simulink model "mech_sticky_box"  (Simulink 7.1)
settings: Solver=ode23t  StartTime=0.0  StopTime=10  RelTol=1e-4  AbsTol=1e-7
libraries: mblibv1 x11, mech_friction x2
Description:
  | Sticky Sliding Boxes
  | 
  | A box sliding on top of another box with sticky friction.
  | 
  | This model demonstrates the use of a stiction actuator. It adds stiction between three boxes on their contacting surfaces. The bottom box is motion-actuated. The velocity plots show periods of zero velocity, indicating locking.
settings Model: Creator=arnav  LastModifiedBy=batserve  ExtModeAutoUpdateStatusClock=off
settings SolverCC: MaxConsecutiveMinStep=10  SolverResetMethod=Robust
settings DataIOCC: OutputOption=SpecifiedOutputTimes  OutputTimes=linspace(0,10,200)  Refine=5
settings OptimizationCC: InlineInvariantSignals=on  BufferReusableBoundary=off
settings DebuggingCC: AlgebraicLoopMsg=none  SaveWithParameterizedLinksMsg=none  SignalResolutionControl=TryResolveAllWithWarning  SolverPrmCheckMsg=none  MultiTaskDSMMsg=warning  MultiTaskCondExecSysMsg=none  SigSpecEnsureSampleTimeMsg=none  UnconnectedInputMsg=none  UnconnectedOutputMsg=none  BusObjectLabelMismatch=none  StrictBusMsg=None
settings HardwareCC: TargetBitPerLong=64  TargetEndianess=LittleEndian  TargetWordSize=64  TargetHWDeviceType=MATLAB Host  ProdEqTarget=off
settings RTWCC: SystemTargetFile=rsim.tlc  TemplateMakefile=rsim_default_tmf  Description=Rapid Simulation Target  ProcessScript=rsim_make_rtw_hook  IncludeERTFirstTime=on
settings RSimTargetCC: TargetFcnLib=ansi_tfl_tmw.mat  TargetFunctionLibrary=ANSI_C  IsPILTarget=off  EnableShiftOperators=on  PortableWordSizes=off
settings SimMechanicsCC: WarnOnRedundantConstraints=off  VisOnUpdateDiagram=on  VisDuringSimulation=on  VisConfigFile=mech_sticky_box.mat

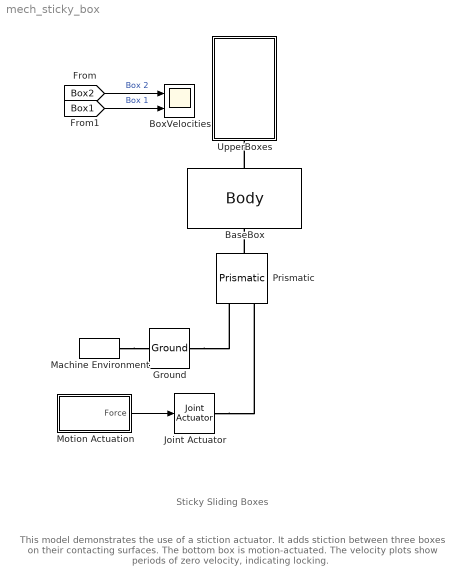
== system mech_sticky_box ==
  note: This model demonstrates the use of a stiction actuator.
      | It adds stiction between three boxes on their contacting surfaces.
      | The bottom box is motion-actuated. The velocity plots show periods
      | of zero velocity, indicating locking.
  note: Sticky Sliding Boxes
  BaseBox : mblibv1/Bodies/Body  Orientation=up  DialogController=MECH.DynMechDlgSource  PhysicalDomain=mechanical  SubClassName=Unknown  LeftPortType=workingframe  RightPortType=workingframe  LConnTagsString=CS1  RConnTagsString=CS2  DialogClass=MechanicalBodyBlock  Mass=1  MassUnits=kg  InertiaUnits=kg*m^2  Inertia=[1 0 0;0 1.9 0;0 0 1]  Shape=Cylinder  ShapeDims=[1 1]  ShapeUnits=m  ShapeUse=false  Density=1  DensityUnits=kg/m^3  DensityUse=false  GraphicsMode=1  BodyColor=[0.5 0.5 0.5]  GraphicsObj=[]  AttachedToCS=1  CG=Left$CG$[0 0.5 0]$CS1$CS1$m$[0 0 0]$Euler X-Y-Z$deg$WORLD$false  WorkingFrames=Left$CS1$[0 0 0]$ADJOINING$ADJOINING$m$[0 0 0]$Euler X-Y-Z$deg$WORLD$true#Right$CS2$[0 1 0]$CS1$CS1$m$[0 0 0]$Euler X-Y-Z$deg$WORLD$true#Right$CS3$[-2 0 2]$CS1$CS1$m$[0 0 0]$Euler X-Y-Z$deg$WORLD$false#Right$CS7$[0 1 0]$CS3$CS3$m$[0 0 0]$Euler X-Y-Z$deg$WORLD$false#Right$CS4$[2 0 2]$CS1$CS1$m$[0 0 0]$Euler X-Y-Z$deg$WORLD$false#Right$CS8$[0 1 0]$CS4$CS4$m$[0 0 0]$Euler X-Y-Z$deg$WORLD$false#Right$CS5$[2 0 -2]$CS1$CS1$m$[0 0 0]$Euler X-Y-Z$deg$WORLD$false#Right$CS9$[0 1 0]$CS5$CS5$m$[0 0 0]$Euler X-Y-Z$deg$WORLD$false#Right$CS6$[-2 0 -2]$CS1$CS1$m$[0 0 0]$Euler X-Y-Z$deg$WORLD$false#Right$CS10$[0 1 0]$CS6$CS6$m$[0 0 0]$Euler X-Y-Z$deg$WORLD$false  CGPos=[0 0.5 0]  CGRot=[0 0 0]  CS0Pos=[]  CS0Rot=[]  CS1Pos=[0 0 0]  CS1Rot=[0 0 0]  CS2Pos=[0 1 0]  CS2Rot=[0 0 0]  CS3Pos=[-2 0 2]  CS3Rot=[0 0 0]  CS4Pos=[2 0 2]  CS4Rot=[0 0 0]  CS5Pos=[2 0 -2]  CS5Rot=[0 0 0]  CS6Pos=[-2 0 -2]  CS6Rot=[0 0 0]  CS7Pos=[0 1 0]  CS7Rot=[0 0 0]  CS8Pos=[0 1 0]  CS8Rot=[0 0 0]  CS9Pos=[0 1 0]  CS9Rot=[0 0 0]  CS10Pos=[0 1 0]  CS10Rot=[0 0 0]  CS11Pos=[]  CS11Rot=[]  CS12Pos=[]  CS12Rot=[]  CS13Pos=[]  CS13Rot=[]  CS14Pos=[]  CS14Rot=[]  CS15Pos=[]  CS15Rot=[]  CS16Pos=[]  CS16Rot=[]  CS17Pos=[]  CS17Rot=[]  CS18Pos=[]  CS18Rot=[]  CS19Pos=[]  CS19Rot=[]  CS20Pos=[]  CS20Rot=[]
  BoxVelocities : Scope  NumInputPorts=2
      settings: TimeRange=10  YMin=-0.4~-1.5  YMax=0.4~1.5
  Ground : mblibv1/Bodies/Ground  DialogController=MECH.DynMechDlgSource  SystemSampleTime=-1  LeftPortType=env  RightPortType=workingframe  PhysicalDomain=Mechanical  DialogClass=GroundBlock  CoordPosition=[0 0 0]  CoordPositionUnits=m  StateVectorMgrId=-1  MachineId=[0 0]  ShowEnvPort=on
  Joint Actuator : mblibv1/Sensors &  Actuators/Joint Actuator  DialogController=MECH.DynMechDlgSource  SystemSampleTime=-1  PhysicalDomain=Mechanical  PortType=blob  ActuationStyle=Force  AngleUnits=deg  ArcVelocityUnits=deg/s  ArcAccelerationUnits=deg/s^2  CoordPositionUnits=m  VelocityUnits=m/s  AccelerationUnits=m/s^2  ForceUnits=N  TorqueUnits=N*m  ActiveIO=on  Width=1  DialogClass=MechanicalActuatorBlock  Primitive=P1  ReferenceFrame=Absolute (INERTIAL)
  Machine Environment : mblibv1/Bodies/Machine Environment  Tag=Factory ground  DialogController=MECH.DialogSource  SystemSampleTime=-1  PortType=env  PhysicalDomain=Mechanical  DialogTemplateClass=MECH.MachineEnvironment  SyncWhenCopied=off  Gravity=[0 -9.81 0]  GravityUnits=m/s^2  GravityAsSignal=off  Dimensionality=Auto-detect  AnalysisType=Forward dynamics  LinearAssemblyTolerance=1e-3  LinearAssemblyToleranceUnits=m  AngularAssemblyTolerance=1e-3  AngularAssemblyToleranceUnits=rad  ConstraintSolverType=Stabilizing  ConstraintRelTolerance=1e-4  ConstraintAbsTolerance=1e-4  UseRobustSingularityHandling=off  RedundancyAnalysisToleranceType=Automatically select tolerance  RedundancyAnalysisTolerance=1e-14  StatePerturbationType=Fixed  PerturbationSize=1e-5  VisualizeMachine=on
  Motion Actuation : Subsystem
  Prismatic : mblibv1/Joints/Prismatic  Orientation=up  DialogController=MECH.DynMechDlgSource  PhysicalDomain=mechanical  SubClassName=Unknown  LeftPortType=blob  RightPortType=blob  LConnTagsString=__newl0|SA1  RConnTagsString=__newr0  NumSAPorts=1  CutJoint=off  MarkAsCut=off  Primitives=prismatic  PrimitiveProps=P1$World$[1 0 0]$prismatic  DialogClass=JointBlock  P1Axis=[1 0 0]
  UpperBoxes : Subsystem  Orientation=up
  wires:
  Motion Actuation/1(Force) -> Joint Actuator/1
  [Box2] -> BoxVelocities/1  "Box 2"
  [Box1] -> BoxVelocities/2  "Box 1"
  connections:
  Machine Environment/RConn1 -- Ground/LConn1
  Ground/RConn1 -- Prismatic/LConn1
  Prismatic/RConn1 -- BaseBox/LConn1
  BaseBox/RConn1 -- UpperBoxes/LConn1
  Joint Actuator/RConn1 -- Prismatic/LConn2

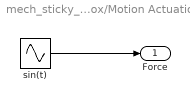
== system mech_sticky_box/Motion Actuation ==
  sin(t) : Sin  Amplitude=7.9  Frequency=3  SampleTime=0
  Force : Outport  OutDataType=sfix(16)  OutScaling=2^0
  wires:
  sin(t)/1 -> Force/1

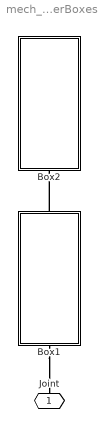
== system mech_sticky_box/UpperBoxes ==
  Box1 : Subsystem  Orientation=up
  Box2 : Subsystem  Orientation=up
  Joint : PMIOPort  Orientation=up  Port=1  Side=Left
  connections:
  Box1/LConn1 -- Joint/RConn1
  Box1/RConn1 -- Box2/LConn1

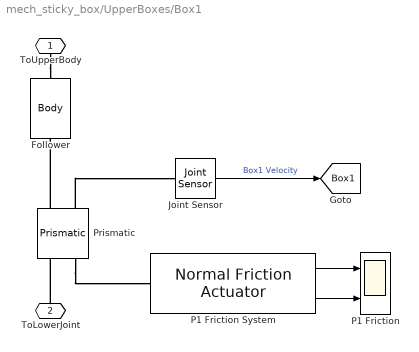
== system mech_sticky_box/UpperBoxes/Box1 ==
  Follower : mblibv1/Bodies/Body  Orientation=up  DialogController=MECH.DynMechDlgSource  PhysicalDomain=mechanical  SubClassName=Unknown  LeftPortType=workingframe  RightPortType=workingframe  LConnTagsString=CS1  RConnTagsString=CS2  DialogClass=MechanicalBodyBlock  Mass=1  MassUnits=kg  InertiaUnits=kg*m^2  Inertia=[1 0 0;0 1.9 0;0 0 1]  Shape=Cylinder  ShapeDims=[1 1]  ShapeUnits=m  ShapeUse=false  Density=1  DensityUnits=kg/m^3  DensityUse=false  GraphicsMode=1  BodyColor=[0.5 0.5 0.5]  GraphicsObj=[]  AttachedToCS=1  CG=Left$CG$[0 0.5 0]$CS1$CS1$m$[0 0 0]$Euler X-Y-Z$deg$WORLD$false  WorkingFrames=Left$CS1$[0 0 0]$ADJOINING$ADJOINING$m$[0 0 0]$Euler X-Y-Z$deg$WORLD$true#Right$CS2$[0 1 0]$CS1$CS1$m$[0 0 0]$Euler X-Y-Z$deg$WORLD$true#Right$CS3$[-2 0 2]$CS1$CS1$m$[0 0 0]$Euler X-Y-Z$deg$WORLD$false#Right$CS7$[0 1 0]$CS3$CS3$m$[0 0 0]$Euler X-Y-Z$deg$WORLD$false#Right$CS4$[2 0 2]$CS1$CS1$m$[0 0 0]$Euler X-Y-Z$deg$WORLD$false#Right$CS8$[0 1 0]$CS4$CS4$m$[0 0 0]$Euler X-Y-Z$deg$WORLD$false#Right$CS5$[2 0 -2]$CS1$CS1$m$[0 0 0]$Euler X-Y-Z$deg$WORLD$false#Right$CS9$[0 1 0]$CS5$CS5$m$[0 0 0]$Euler X-Y-Z$deg$WORLD$false#Right$CS6$[-2 0 -2]$CS1$CS1$m$[0 0 0]$Euler X-Y-Z$deg$WORLD$false#Right$CS10$[0 1 0]$CS6$CS6$m$[0 0 0]$Euler X-Y-Z$deg$WORLD$false  CGPos=[0 0.5 0]  CGRot=[0 0 0]  CS0Pos=[]  CS0Rot=[]  CS1Pos=[0 0 0]  CS1Rot=[0 0 0]  CS2Pos=[0 1 0]  CS2Rot=[0 0 0]  CS3Pos=[-2 0 2]  CS3Rot=[0 0 0]  CS4Pos=[2 0 2]  CS4Rot=[0 0 0]  CS5Pos=[2 0 -2]  CS5Rot=[0 0 0]  CS6Pos=[-2 0 -2]  CS6Rot=[0 0 0]  CS7Pos=[0 1 0]  CS7Rot=[0 0 0]  CS8Pos=[0 1 0]  CS8Rot=[0 0 0]  CS9Pos=[0 1 0]  CS9Rot=[0 0 0]  CS10Pos=[0 1 0]  CS10Rot=[0 0 0]  CS11Pos=[]  CS11Rot=[]  CS12Pos=[]  CS12Rot=[]  CS13Pos=[]  CS13Rot=[]  CS14Pos=[]  CS14Rot=[]  CS15Pos=[]  CS15Rot=[]  CS16Pos=[]  CS16Rot=[]  CS17Pos=[]  CS17Rot=[]  CS18Pos=[]  CS18Rot=[]  CS19Pos=[]  CS19Rot=[]  CS20Pos=[]  CS20Rot=[]
  Joint Sensor : mblibv1/Sensors &  Actuators/Joint Sensor  DialogController=MECH.DynMechDlgSource  SystemSampleTime=-1  PhysicalDomain=Mechanical  PortType=blob  Muxed=on  Pose=off  Angle=on  AngleUnits=deg  ArcVelocity=off  ArcVelocityUnits=deg/s  ArcAcceleration=off  ArcAccelerationUnits=deg/s^2  CoordPosition=off  CoordPositionUnits=m  Velocity=on  VelocityUnits=m/s  Acceleration=off  AccelerationUnits=m/s^2  Quaternion=on  QuaternionDT=off  QuaternionDDT=off  QuaternionUnits=off  OutputVector=[ 1 ]  ActiveIO=on  Width=1  DialogClass=MechanicalSensorBlock  Primitive=P1  Force=off  ForceUnits=N  Torque=off  TorqueUnits=N*m  ReferenceFrame=Absolute (INERTIAL)  ReactionSensedSide=Base  ReactionReferenceFrame=Absolute (World)  ReactionForce=off  ReactionForceUnits=N  ReactionMoment=off  ReactionMomentUnits=N*m
  P1 Friction : Scope  NumInputPorts=2
      settings: TimeRange=10  YMin=-50~-10  YMax=50~0
  P1 Friction System : mech_friction/Normal Friction Actuator  SystemSampleTime=-1  Ckinetic=0.1  staticFF=1.65  Csforward=0.055  Csreverse=0.055  sExtActuation=off  sForces=on  primitive=P1
  Prismatic : mblibv1/Joints/Prismatic  Orientation=up  DialogController=MECH.DynMechDlgSource  PhysicalDomain=mechanical  SubClassName=Unknown  LeftPortType=blob  RightPortType=blob  LConnTagsString=__newl0|SA1  RConnTagsString=__newr0|SA1  NumSAPorts=2  CutJoint=off  MarkAsCut=off  Primitives=prismatic  PrimitiveProps=P1$World$[1 0 0]$prismatic  DialogClass=JointBlock  P1Axis=[1 0 0]
  ToUpperBody : PMIOPort  Orientation=down  Port=1  Side=Right
  ToLowerJoint : PMIOPort  Orientation=up  Port=2  Side=Left
  tag scope: Box1=global
  wires:
  P1 Friction System/1 -> P1 Friction/1
  P1 Friction System/2 -> P1 Friction/2
  Joint Sensor/1 -> [Box1]  "Box1 Velocity"
  connections:
  Prismatic/RConn1 -- Follower/LConn1
  Prismatic/RConn2 -- Joint Sensor/LConn1
  Prismatic/LConn2 -- P1 Friction System/LConn1
  ToUpperBody/RConn1 -- Follower/RConn1
  ToLowerJoint/RConn1 -- Prismatic/LConn1

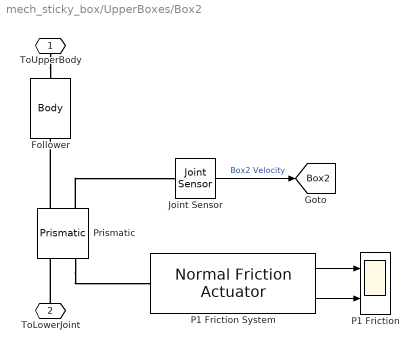
== system mech_sticky_box/UpperBoxes/Box2 ==
  Follower : mblibv1/Bodies/Body  Orientation=up  DialogController=MECH.DynMechDlgSource  PhysicalDomain=mechanical  SubClassName=Unknown  LeftPortType=workingframe  RightPortType=workingframe  LConnTagsString=CS1  RConnTagsString=CS2  DialogClass=MechanicalBodyBlock  Mass=2  MassUnits=kg  InertiaUnits=kg*m^2  Inertia=[1 0 0;0 1.9 0;0 0 1]  Shape=Cylinder  ShapeDims=[1 1]  ShapeUnits=m  ShapeUse=false  Density=1  DensityUnits=kg/m^3  DensityUse=false  GraphicsMode=1  BodyColor=[0.5 0.5 0.5]  GraphicsObj=[]  AttachedToCS=1  CG=Left$CG$[0 0.4 0]$CS1$CS1$m$[0 0 0]$Euler X-Y-Z$deg$WORLD$false  WorkingFrames=Left$CS1$[0 0 0]$ADJOINING$ADJOINING$m$[0 0 0]$Euler X-Y-Z$deg$WORLD$true#Right$CS2$[0 1 0]$CS1$CS1$m$[0 0 0]$Euler X-Y-Z$deg$WORLD$true#Right$CS3$[-2 0 2]$CS1$CS1$m$[0 0 0]$Euler X-Y-Z$deg$WORLD$false#Right$CS7$[0 1 0]$CS3$CS3$m$[0 0 0]$Euler X-Y-Z$deg$WORLD$false#Right$CS4$[2 0 2]$CS1$CS1$m$[0 0 0]$Euler X-Y-Z$deg$WORLD$false#Right$CS8$[0 1 0]$CS4$CS4$m$[0 0 0]$Euler X-Y-Z$deg$WORLD$false#Right$CS5$[2 0 -2]$CS1$CS1$m$[0 0 0]$Euler X-Y-Z$deg$WORLD$false#Right$CS9$[0 1 0]$CS5$CS5$m$[0 0 0]$Euler X-Y-Z$deg$WORLD$false#Right$CS6$[-2 0 -2]$CS1$CS1$m$[0 0 0]$Euler X-Y-Z$deg$WORLD$false#Right$CS10$[0 1 0]$CS6$CS6$m$[0 0 0]$Euler X-Y-Z$deg$WORLD$false  CGPos=[0 0.4 0]  CGRot=[0 0 0]  CS0Pos=[]  CS0Rot=[]  CS1Pos=[0 0 0]  CS1Rot=[0 0 0]  CS2Pos=[0 1 0]  CS2Rot=[0 0 0]  CS3Pos=[-2 0 2]  CS3Rot=[0 0 0]  CS4Pos=[2 0 2]  CS4Rot=[0 0 0]  CS5Pos=[2 0 -2]  CS5Rot=[0 0 0]  CS6Pos=[-2 0 -2]  CS6Rot=[0 0 0]  CS7Pos=[0 1 0]  CS7Rot=[0 0 0]  CS8Pos=[0 1 0]  CS8Rot=[0 0 0]  CS9Pos=[0 1 0]  CS9Rot=[0 0 0]  CS10Pos=[0 1 0]  CS10Rot=[0 0 0]  CS11Pos=[]  CS11Rot=[]  CS12Pos=[]  CS12Rot=[]  CS13Pos=[]  CS13Rot=[]  CS14Pos=[]  CS14Rot=[]  CS15Pos=[]  CS15Rot=[]  CS16Pos=[]  CS16Rot=[]  CS17Pos=[]  CS17Rot=[]  CS18Pos=[]  CS18Rot=[]  CS19Pos=[]  CS19Rot=[]  CS20Pos=[]  CS20Rot=[]
  Joint Sensor : mblibv1/Sensors &  Actuators/Joint Sensor  DialogController=MECH.DynMechDlgSource  SystemSampleTime=-1  PhysicalDomain=Mechanical  PortType=blob  Muxed=on  Pose=off  Angle=on  AngleUnits=deg  ArcVelocity=off  ArcVelocityUnits=deg/s  ArcAcceleration=off  ArcAccelerationUnits=deg/s^2  CoordPosition=off  CoordPositionUnits=m  Velocity=on  VelocityUnits=m/s  Acceleration=off  AccelerationUnits=m/s^2  Quaternion=on  QuaternionDT=off  QuaternionDDT=off  QuaternionUnits=off  OutputVector=[ 1 ]  ActiveIO=on  Width=1  DialogClass=MechanicalSensorBlock  Primitive=P1  Force=off  ForceUnits=N  Torque=off  TorqueUnits=N*m  ReferenceFrame=Absolute (INERTIAL)  ReactionSensedSide=Base  ReactionReferenceFrame=Absolute (World)  ReactionForce=off  ReactionForceUnits=N  ReactionMoment=off  ReactionMomentUnits=N*m
  P1 Friction : Scope  NumInputPorts=2
      settings: TimeRange=10  YMin=-50~-10  YMax=50~0
  P1 Friction System : mech_friction/Normal Friction Actuator  SystemSampleTime=-1  Ckinetic=0.1  staticFF=1.63  Csforward=0.055  Csreverse=0.055  sExtActuation=off  sForces=on  primitive=P1
  Prismatic : mblibv1/Joints/Prismatic  Orientation=up  DialogController=MECH.DynMechDlgSource  PhysicalDomain=mechanical  SubClassName=Unknown  LeftPortType=blob  RightPortType=blob  LConnTagsString=__newl0|SA1  RConnTagsString=__newr0|SA1  NumSAPorts=2  CutJoint=off  MarkAsCut=off  Primitives=prismatic  PrimitiveProps=P1$World$[1 0 0]$prismatic  DialogClass=JointBlock  P1Axis=[1 0 0]
  ToUpperBody : PMIOPort  Orientation=down  Port=1  Side=Right
  ToLowerJoint : PMIOPort  Orientation=up  Port=2  Side=Left
  tag scope: Box2=global
  wires:
  Joint Sensor/1 -> [Box2]  "Box2 Velocity"
  P1 Friction System/2 -> P1 Friction/2
  P1 Friction System/1 -> P1 Friction/1
  connections:
  ToLowerJoint/RConn1 -- Prismatic/LConn1
  ToUpperBody/RConn1 -- Follower/RConn1
  Prismatic/LConn2 -- P1 Friction System/LConn1
  Prismatic/RConn2 -- Joint Sensor/LConn1
  Prismatic/RConn1 -- Follower/LConn1
